simulink model "Main_Sim_FlatSat"  (R2018b)
settings: Solver=FixedStepAuto  StartTime=0.0  StopTime=600  FixedStep=simParams.sample_time_s  RelTol=1e-3  EnableMultiTasking=on
libraries: Environment_lib x1, FlatSatRead_lib x1, FlatSatWrite_lib x1, Sensors_Lib x1, satelliteDynamics_lib x1
settings Model: Creator=devantormey  LastModifiedBy=Taylor
settings OptimizationCC: DefaultParameterBehavior=Inlined  UseDivisionForNetSlopeComputation=on  UseFloatMulNetSlope=on  InlineInvariantSignals=on  PassReuseOutputArgsAs=Individual arguments  ZeroExternalMemoryAtStartup=off  ZeroInternalMemoryAtStartup=off  NoFixptDivByZeroProtection=on  EfficientFloat2IntCast=on  LifeSpan=1  OptimizeBlockOrder=speed  DifferentSizesBufferReuse=on
settings DebuggingCC: ParameterTunabilityLossMsg=error  BusObjectLabelMismatch=error  SFUnexpectedBacktrackingDiag=warning  SFNoUnconditionalDefaultTransitionDiag=warning
settings HardwareCC: ProdBitPerPointer=32  ProdBitPerSizeT=32  ProdBitPerPtrDiffT=32  ProdLargestAtomicInteger=Long  ProdLargestAtomicFloat=Double  ProdWordSize=32  ProdLongLongMode=on  ProdHWDeviceType=NXP->Cortex-M4
settings SFSimCC: SimUseLocalCustomCode=off  MATLABDynamicMemAlloc=off
settings RTWCC: SystemTargetFile=ert.tlc  TemplateMakefile=ert_default_tmf  GenerateReport=on  RTWUseLocalCustomCode=off  IncludeHyperlinkInReport=on  LaunchReport=on  GenerateTraceInfo=on  GenerateTraceReport=on  GenerateTraceReportSl=on  GenerateTraceReportSf=on  GenerateTraceReportEml=on  GenerateCodeMetricsReport=on
settings CodeAppCC: ForceParamTrailComments=on  IgnoreCustomStorageClasses=off  OperatorAnnotations=on  SimulinkDataObjDesc=on  SFDataObjDesc=on  CustomSymbolStrGlobalVar=rt$N$M  CustomSymbolStrType=$N$M  CustomSymbolStrFcn=$N$M$F  CustomSymbolStrMacro=$N$M  InsertBlockDesc=on
settings ERTTargetCC: GenerateSampleERTMain=on  IncludeMdlTerminateFcn=off  CombineSignalStateStructs=on  SupportComplex=off  SupportContinuousTime=on  SupportNonInlinedSFcns=on  InlinedParameterPlacement=NonHierarchical  ERTCustomFileTemplate=example_file_process.tlc
settings ConfigComp: CovMetricSettings=dw  CovHtmlReporting=on  CovSaveCumulativeToWorkspaceVar=on  CovSaveSingleToWorkspaceVar=on  CovExternalEMLEnable=off

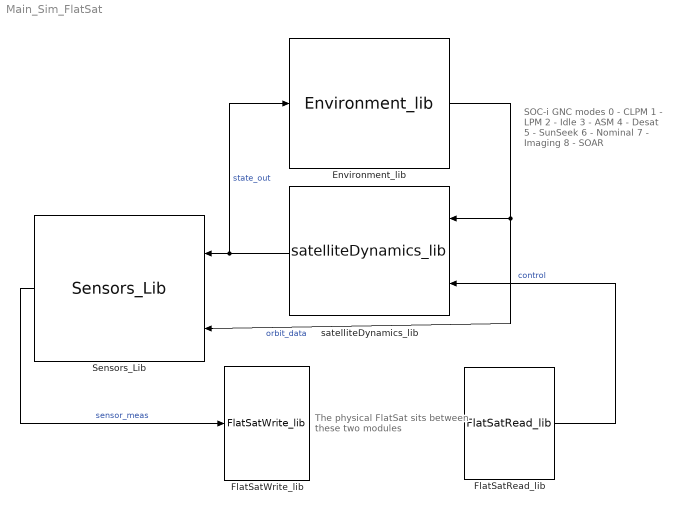
== system Main_Sim_FlatSat ==
  note: The physical FlatSat sits
      | between these two modules
  note: SOC-i GNC modes
      | 0 - CLPM
      | 1 - LPM
      | 2 - Idle
      | 3 - ASM
      | 4 - Desat
      | 5 - SunSeek
      | 6 - Nominal
      | 7 - Imaging
      | 8 - SOAR
  Environment_lib : Environment_lib/Environment_lib  SystemSampleTime=-1
  FlatSatRead_lib : FlatSatRead_lib/FlatSatRead_lib  SystemSampleTime=-1
  FlatSatWrite_lib : FlatSatWrite_lib/FlatSatWrite_lib  SystemSampleTime=-1
  Sensors_Lib : Sensors_Lib/Sensors_Lib  SystemSampleTime=-1
      link override magnetometer_array/magnetometer_lib2: id_s=3
  satelliteDynamics_lib : satelliteDynamics_lib/satelliteDynamics_lib  SystemSampleTime=-1
  wires:
  Sensors_Lib/1 -> FlatSatWrite_lib/1  "sensor_meas"
  satelliteDynamics_lib/1 -> Sensors_Lib/1, Environment_lib/1  "state_out"
  Environment_lib/1 -> Sensors_Lib/2, satelliteDynamics_lib/1  "orbit_data"
  FlatSatRead_lib/1 -> satelliteDynamics_lib/2  "control"
